simulink model "mainModel_matlab2013b"  (R2013b)
settings: Solver=ode45  SolverMode=SingleTasking  StartTime=0.0  StopTime=1000  RelTol=1e-5
settings Model: CovMetricSettings=dwe  CovHtmlReporting=off  covSaveCumulativeToWorkspaceVar=off  CovSaveSingleToWorkspaceVar=off  CovExternalEMLEnable=on  Creator=manoj  LastModifiedBy=manoj
settings DataIOCC: LimitDataPoints=off  SaveFormat=StructureWithTime
settings DebuggingCC: UnderspecifiedInitializationDetection=Simplified  MergeDetectMultiDrivingBlocksExec=error  SolverPrmCheckMsg=none  FrameProcessingCompatibilityMsg=error  SFUnexpectedBacktrackingDiag=error  SFNoUnconditionalDefaultTransitionDiag=error
settings HardwareCC: ProdBitPerPointer=64  ProdLargestAtomicFloat=Float  ProdIntDivRoundTo=Zero  ProdEndianess=LittleEndian  ProdHWDeviceType=Specified
settings ModelReferenceCC: PropagateSignalLabelsOutOfModel=on
settings GRTTargetCC: CodeReplacementLibrary=C99 (ISO)  GeneratePreprocessorConditionals=Use local settings

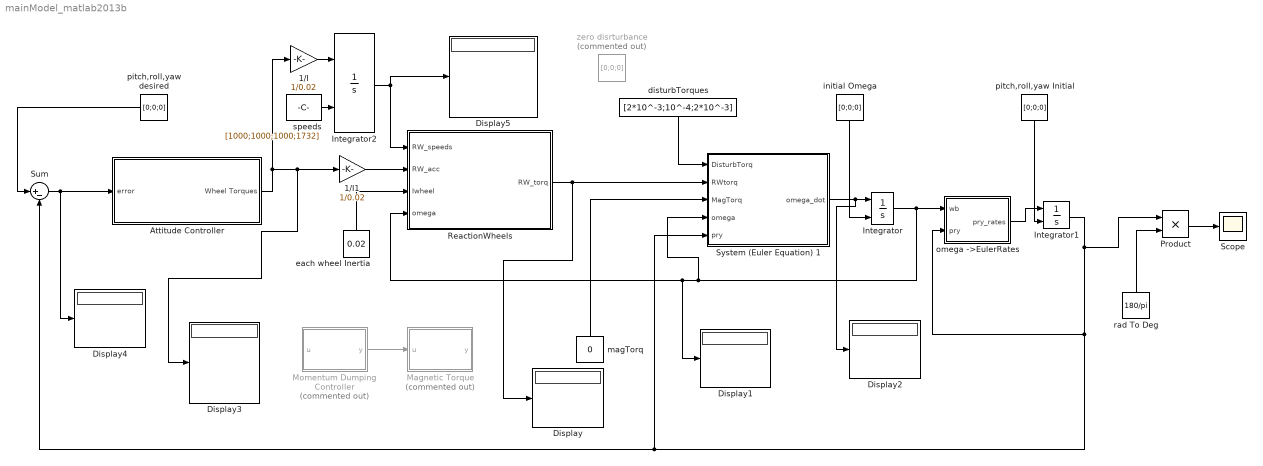
== system mainModel_matlab2013b ==
  1/I : Gain  Gain=1/0.02
  1/I1 : Gain  Gain=1/0.02
  Attitude Controller : Subsystem
  Display{,1..5} (6 alike) : Display
  Integrator : Integrator  InitialConditionSource=external
  Integrator1 : Integrator  InitialConditionSource=external
  Integrator2 : Integrator  InitialConditionSource=external  LimitOutput=on  UpperSaturationLimit=2000  LowerSaturationLimit=100
  "Magnetic Torque " : MATLAB Function  Commented=on  TreatAsAtomicUnit=on
      settings: PermitHierarchicalResolution=ParametersOnly
  Momentum Dumping Controller : MATLAB Function  Commented=on  TreatAsAtomicUnit=on
      settings: PermitHierarchicalResolution=ParametersOnly
  Product : Product
  ReactionWheels : MATLAB Function  TreatAsAtomicUnit=on
      settings: PermitHierarchicalResolution=ParametersOnly
  Scope : Scope
      settings: TimeRange=auto  ShowLegends=on  MaxDataPoints=5000  SaveToWorkspace=off  SaveName=ScopeData  YMin=-4.33068  YMax=38.97609  SampleTime=-1
  Sum : Sum  Inputs=|+-
  System (Euler Equation) 1 : MATLAB Function  TreatAsAtomicUnit=on
      settings: PermitHierarchicalResolution=ParametersOnly
  disturbTorques : Constant  Value=[2*10^-3;10^-4;2*10^-3]
  each wheel Inertia : Constant  Value=0.02
  initial Omega : Constant  Value=[0;0;0]
  "magTorq " : Constant  Value=0
  omega ->EulerRates : MATLAB Function  TreatAsAtomicUnit=on
      settings: PermitHierarchicalResolution=ParametersOnly
  pitch,roll,yaw Initial : Constant  Value=[0;0;0]
  pitch,roll,yaw desired : Constant  Value=[0;0;0]
  rad To Deg : Constant  Value=180/pi
  speeds : Constant  Value=[1000;1000;1000;1732]
  "zero disrturbance " : Constant  Commented=on  Value=[0;0;0]
  wires:
  Attitude Controller/1(Wheel Torques) -> 1/I/1, Display3/1, 1/I1/1
  Momentum Dumping Controller/1(y) -> "Magnetic Torque "/1(u)
  each wheel Inertia/1 -> ReactionWheels/3(Iwheel)
  Integrator2/1 -> ReactionWheels/1(RW_speeds), Display5/1
  speeds/1 -> Integrator2/2
  Integrator/1 -> System (Euler Equation) 1/4(omega), Display1/1, ReactionWheels/4(omega), omega ->EulerRates/1(wb)
  Integrator1/1 -> Product/1, omega ->EulerRates/2(pry), System (Euler Equation) 1/5(pry), Sum/2
  ReactionWheels/1(RW_torq) -> System (Euler Equation) 1/2(RWtorq), Display/1
  omega ->EulerRates/1(pry_rates) -> Integrator1/1
  "magTorq "/1 -> System (Euler Equation) 1/3(MagTorq)
  initial Omega/1 -> Integrator/2
  pitch,roll,yaw Initial/1 -> Integrator1/2
  Product/1 -> Scope/1
  rad To Deg/1 -> Product/2
  System (Euler Equation) 1/1(omega_dot) -> Display2/1, Integrator/1
  disturbTorques/1 -> System (Euler Equation) 1/1(DisturbTorq)
  1/I/1 -> Integrator2/1
  pitch,roll,yaw desired/1 -> Sum/1
  Sum/1 -> Display4/1, Attitude Controller/1(error)
  1/I1/1 -> ReactionWheels/2(RW_acc)

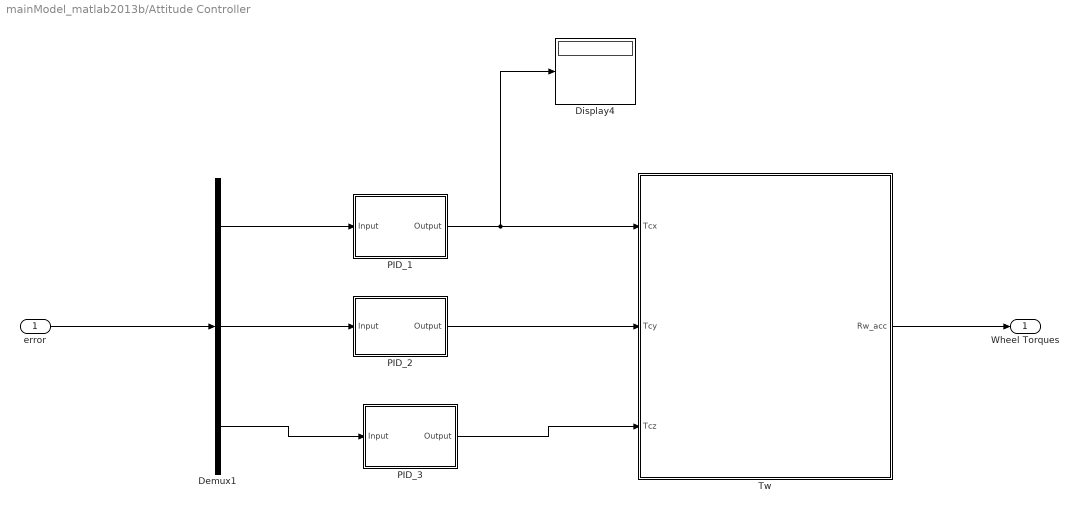
== system mainModel_matlab2013b/Attitude Controller ==
  error : Inport
  Demux1 : Demux  Outputs=3
  Display4 : Display
  PID_1 : Subsystem
  PID_2 : Subsystem
  PID_3 : Subsystem
  "Tw " : MATLAB Function  TreatAsAtomicUnit=on
      settings: PermitHierarchicalResolution=ParametersOnly
  Wheel Torques : Outport
  wires:
  error/1 -> Demux1/1
  "Tw "/1(Rw_acc) -> Wheel Torques/1
  Demux1/1 -> PID_1/1(Input)
  PID_1/1(Output) -> Display4/1, "Tw "/1(Tcx)
  Demux1/2 -> PID_2/1(Input)
  PID_2/1(Output) -> "Tw "/2(Tcy)
  Demux1/3 -> PID_3/1(Input)
  PID_3/1(Output) -> "Tw "/3(Tcz)

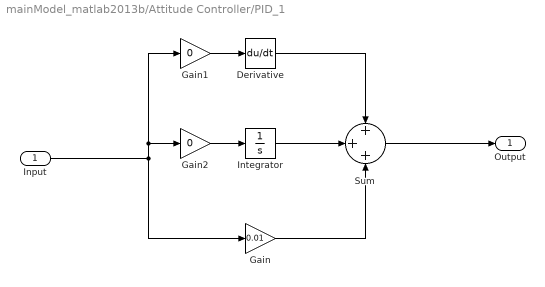
== system mainModel_matlab2013b/Attitude Controller/PID_1 ==
  Input : Inport
  Derivative : Derivative
  Gain : Gain  Gain=0.01
  Gain1 : Gain  Gain=0
  Gain2 : Gain  Gain=0
  Integrator : Integrator
  Sum : Sum  Inputs=+++
  Output : Outport
  wires:
  Gain1/1 -> Derivative/1
  Integrator/1 -> Sum/2
  Sum/1 -> Output/1
  Gain2/1 -> Integrator/1
  Derivative/1 -> Sum/1
  Gain/1 -> Sum/3
  Input/1 -> Gain1/1, Gain2/1, Gain/1

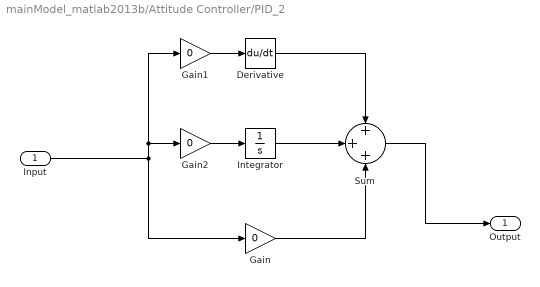
== system mainModel_matlab2013b/Attitude Controller/PID_2 ==
  Input : Inport
  Derivative : Derivative
  Gain : Gain  Gain=0
  Gain1 : Gain  Gain=0
  Gain2 : Gain  Gain=0
  Integrator : Integrator
  Sum : Sum  Inputs=+++
  Output : Outport
  wires:
  Gain1/1 -> Derivative/1
  Integrator/1 -> Sum/2
  Sum/1 -> Output/1
  Gain2/1 -> Integrator/1
  Derivative/1 -> Sum/1
  Gain/1 -> Sum/3
  Input/1 -> Gain1/1, Gain2/1, Gain/1

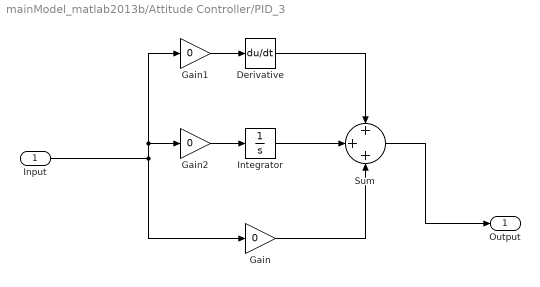
== system mainModel_matlab2013b/Attitude Controller/PID_3 ==
  Input : Inport
  Derivative : Derivative
  Gain : Gain  Gain=0
  Gain1 : Gain  Gain=0
  Gain2 : Gain  Gain=0
  Integrator : Integrator
  Sum : Sum  Inputs=+++
  Output : Outport
  wires:
  Gain1/1 -> Derivative/1
  Integrator/1 -> Sum/2
  Sum/1 -> Output/1
  Gain2/1 -> Integrator/1
  Derivative/1 -> Sum/1
  Gain/1 -> Sum/3
  Input/1 -> Gain1/1, Gain2/1, Gain/1

== matlab function mainModel_matlab2013b/Attitude Controller/Tw  ==
  data: Tcx input; Tcy input; Rw_acc output; Tcz input
function Rw_acc = fcn(Tcx,Tcy,Tcz)
%Rw_acc=[0;0;0;0]; %no controller for now. This acceleration correspond
% to the rate of change in speed of each wheel. wheel speeds are always
% positive buy convention
Tc = [Tcx;Tcy;Tcz];

a = -1/sqrt(3);
b = -1/sqrt(3);
g = -1/sqrt(3);

Conv = [1+b^2+g^2, -a*b,      -a*g;
          -a*b,    1+a^2+g^2,  -b*g;
          -a*g,      -b*g,    1+a^2+b^2;
            a ,        b ,       g];

Conv = 0.5*Conv

Rw_acc = Conv*Tc;
end

== matlab function mainModel_matlab2013b/System (Euler Equation) 1 ==
  data: DisturbTorq input; RWtorq input; omega_dot output; MagTorq input; omega input; pry input
function omega_dot = fcn( DisturbTorq,RWtorq,MagTorq,omega,pry)
%[x,y,z] corresponds to yaw roll and pitch axis!!!
%omega written here is wrt orbit and written in body frame
MOI=[1800 -50 -15;-50 1600 25;-15 25 1200];%momentOfInertia of Satellite(with everything)
%Mass=1600;%kg
p=pry(1);
r=pry(2);
y=pry(3);
Cx=[    1, 0, 0
        0, cos(y), sin(y)
        0, -sin(y), cos(y)];

Cy=[    cos(r), 0, -sin(r);
        0, 1, 0;
        sin(r), 0, cos(r) ];

Cz=[    cos(p), sin(p), 0;
        -sin(p), cos(p), 0;
        0, 0, 1    ];
Cbo=Cx*Cy*Cz; %orbit to body frame matrix adopting 3,2,1 convention on (x,y,z)
Wo=1.0741*10^-3;
temp1=(omega-Cbo*[0;0;Wo]);
temp2=cross(omega,Cbo*[0;0;Wo]);
omega_dot=(MOI)\(DisturbTorq+MagTorq-RWtorq-cross(temp1,MOI*temp1))-temp2;

end

== matlab function mainModel_matlab2013b/Magnetic Torque  ==
  data: u input; y output
function y = fcn(u)

y = u;

== matlab function mainModel_matlab2013b/omega ->EulerRates ==
  data: wb input; pry_rates output; pry input
function pry_rates  = fcn(wb,pry)
%[x,y,z] 3-2-1 rotation, where x=yaw,y=roll,z=pitch axis
% pry-pitch,yaw,roll angles

% Cx=[    1, 0, 0
%         0, cos(yaw), sin(yaw)
%         0, -sin(yaw), cos(yaw)    ];
% 
% Cy=[    cos(roll), 0, -sin(roll);
%         0, 1, 0;
%         sin(roll), 0, cos(roll) ];
% 
% Cz=[    cos(pitch), sin(pitch), 0;
%         -sin(pitch), cos(pitch), 0;
%         0, 0, 1    ];NOT NEEDED HERE BUT CAN BE USED ELSEWHERE IF NEEDEd

%p=pry(1);
r=pry(2);
y=pry(3);
C_pryToOmega=   [   -sin(r),        0,      1
                    cos(r)*sin(y),  cos(y), 0
                    cos(r)*cos(y), -sin(y), 0];
pry_rates=(C_pryToOmega)\wb;

== matlab function mainModel_matlab2013b/ReactionWheels ==
  data: RW_speeds input; RW_acc input; RW_torq output size=3; Iwheel input; omega input
function RW_torq = fcn(RW_speeds,RW_acc,Iwheel,omega)
%For Normal arrangement(not the tetrahedron one)
%RW_acc means acceleration of 4 individual wheel speeds

Torq_acceleration_part=Iwheel*[  RW_acc(1)-1/sqrt(3)*RW_acc(4);
                            RW_acc(2)-1/sqrt(3)*RW_acc(4);
                            RW_acc(3)-1/sqrt(3)*RW_acc(4)  ];
Torq_gyroscopic_part=Iwheel*[ RW_speeds(3)*omega(2)- RW_speeds(2)*omega(3);
                              RW_speeds(1)*omega(3)- RW_speeds(3)*omega(1);
                              RW_speeds(2)*omega(1)- RW_speeds(1)*omega(2)];
RW_torq=Torq_acceleration_part+Torq_gyroscopic_part;%gyroscopic part is actually undesired but still present                            
end

== matlab function mainModel_matlab2013b/Momentum Dumping Controller ==
  data: u input; y output
function y = fcn(u)

y = u;
